simulink library "solar_P"  (R2018b)
settings: Solver=VariableStepAuto  StartTime=0.0  StopTime=10.0  RelTol=1e-3
libraries: vrlib x1
settings Model: Creator=devantormey  LastModifiedBy=devantormey

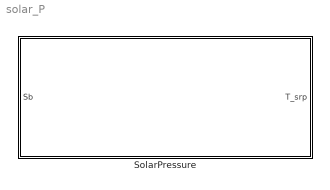
== system solar_P ==
  SolarPressure : Subsystem

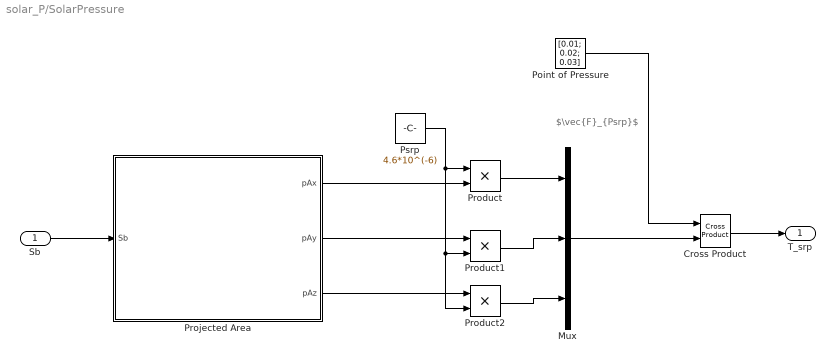
== system solar_P/SolarPressure ==
  note: $\vec{F}_{Psrp}$
  Sb : Inport
  Cross Product : vrlib/Utilities/Cross Product
      settings: SourceProductBaseCode=VR
  Mux : Mux  Inputs=3
  Point of Pressure : Constant  Value=[0.01; 0.02; 0.03]
  Product : Product
  Product1 : Product
  Product2 : Product
  Projected Area : Subsystem
  Psrp : Constant  Value=4.6*10^(-6)
  T_srp : Outport
  wires:
  Sb/1 -> Projected Area/1(Sb)
  Projected Area/1(pAx) -> Product/2
  Psrp/1 -> Product2/2, Product1/2, Product/1
  Projected Area/2(pAy) -> Product1/1
  Projected Area/3(pAz) -> Product2/1
  Product/1 -> Mux/1
  Product1/1 -> Mux/2
  Product2/1 -> Mux/3
  Point of Pressure/1 -> Cross Product/1
  Mux/1 -> Cross Product/2
  Cross Product/1 -> T_srp/1

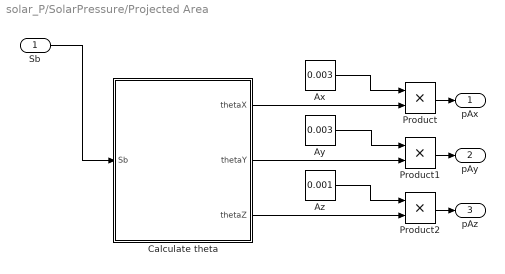
== system solar_P/SolarPressure/Projected Area ==
  Sb : Inport
  Ax : Constant  Value=0.003
  Ay : Constant  Value=0.003
  Az : Constant  Value=0.001
  Calculate theta : MATLAB Function  TreatAsAtomicUnit=on
  Product : Product
  Product1 : Product
  Product2 : Product
  pAx : Outport
  pAy : Outport  Port=2
  pAz : Outport  Port=3
  wires:
  Product1/1 -> pAy/1
  Product2/1 -> pAz/1
  Az/1 -> Product2/1
  Calculate theta/3(thetaZ) -> Product2/2
  Ay/1 -> Product1/1
  Calculate theta/1(thetaX) -> Product/2
  Calculate theta/2(thetaY) -> Product1/2
  Product/1 -> pAx/1
  Sb/1 -> Calculate theta/1(Sb)
  Ax/1 -> Product/1

== matlab function solar_P/SolarPressure/Projected Area/Calculate theta ==
  data: Sb input; thetaX output; thetaY output; thetaZ output
% Author: Devan Tormey
% Date: 2/21/2019
function [thetaX,thetaY,thetaZ] = fcn(Sb)
% Description: This function computes the dot product of the sun vector
% with the appropriate body coordinate vector.
%~~~~~~~~~~~~~ 
%  Variables 
%~~~~~~~~~~~~~~
% Sb - this is the sun vector (calculated elsewhere)
% ThetaXYZ - as these are all unit vectors the dot product produces the
% cosine of the angle in between

    if Sb(1) >= 0 
        thetaX = dot(Sb,[1;0;0]);
    else 
        thetaX = dot(Sb,[-1;0;0]);
    end

    if Sb(2) >= 0 
        thetaY = dot(Sb,[0;1;0]);
    else 
        thetaY = dot(Sb,[0;-1;0]);
    end

    if Sb(3) >= 0 
        thetaZ = dot(Sb,[0;0;1]);
    else 
        thetaZ = dot(Sb,[0;0;-1]);
    end

end
